simulink model "SOE_H2_DRI_plant"  (R2023b)
settings: Solver=ode15s  StartTime=0.0  StopTime=3600*24*8759
values from neighbouring files (symbols this model uses):
  a_b = 6*(1-eps_bed)/(r_p*2)    (= 200)    [H2_DRI_plant_loader.m]
  A_furnace = pi*r_furnace^2    (= 23.7582944428)    [H2_DRI_plant_loader.m]
  A_furnace_pel = A_furnace*(1-eps_bed)    (= 11.8791472214)    [H2_DRI_plant_loader.m]
  A_wall = (2*pi*r_furnace*dz)    (= 1.1674837564)    [H2_DRI_plant_loader.m]
  c_CH4init = interp1([1:1:length(c_CH4init)],c_CH4init, linspace(1,length(c_CH4init),n_furnace))    [H2_DRI_plant_loader.m]    (also in inital_conditions.m = out.CH4_conc.data(end,:); initcond_H2.mat = [9.94099064213e-45 -4.26076213273e-25 -4.27813906239e-25 -4.; initcond_H2_PEM.mat = [4.30667282687e-45 4.29087427587e-45 3.8700760922e-45 3.7994)
  c_Cinit = interp1([1:1:length(c_Cinit)],c_Cinit, linspace(1,length(c_Cinit),n_furnace))    [H2_DRI_plant_loader.m]    (also in inital_conditions.m = out.C_conc.data(end,:); initcond_H2.mat = [1.45956980986e-305 6.99081092012e-307 8.03725154841e-309 -3; initcond_H2_PEM.mat = [1.92191536232e-321 1.91203404941e-321 1.97132192691e-321 1.)
  c_CO2init = interp1([1:1:length(c_CO2init)],c_CO2init, linspace(1,length(c_CO2init),n_furnace))    [H2_DRI_plant_loader.m]    (also in inital_conditions.m = out.CO2_conc.data(end,:); initcond_H2.mat = [1.40671287015e-53 9.99429922421e-25 1.00349747704e-24 1.007; initcond_H2_PEM.mat = [4.30579616214e-45 4.28998535938e-45 3.86916279543e-45 3.798)
  c_COinit = interp1([1:1:length(c_COinit)],c_COinit, linspace(1,length(c_COinit),n_furnace))    [H2_DRI_plant_loader.m]    (also in inital_conditions.m = out.CO_conc.data(end,:); initcond_H2.mat = [8.62168160047e-54 2.62488347241e-25 2.63562031881e-25 2.646; initcond_H2_PEM.mat = [-1.41770643933e-43 -1.41248114323e-43 -1.27321677334e-43 -1)
  c_Fe2O3init = interp1([1:1:length(c_Fe2O3init)],c_Fe2O3init, linspace(1,length(c_Fe2O3init),n_furnace))    [H2_DRI_plant_loader.m]    (also in inital_conditions.m = out.Fe2O3_conc.data(end,:); initcond_H2.mat = [-0.0576294325141 -0.0562977053664 -0.0549879883395 -0.05369; initcond_H2_PEM.mat = [-0.0421766495112 -0.0410731169681 -0.0399918101679 -0.03893)
  c_Fe3O4init = interp1([1:1:length(c_Fe3O4init)],c_Fe3O4init, linspace(1,length(c_Fe3O4init),n_furnace))    [H2_DRI_plant_loader.m]    (also in inital_conditions.m = out.Fe3O4_conc.data(end,:); initcond_H2.mat = [0.0460784397936 0.0452182842983 0.0443654100081 0.043519007; initcond_H2_PEM.mat = [0.0345314201173 0.0338401633931 0.0331554273597 0.032476466)
  c_Feinit = interp1([1:1:length(c_Feinit)],c_Feinit, linspace(1,length(c_Feinit),n_furnace))    [H2_DRI_plant_loader.m]    (also in inital_conditions.m = out.Fe_conc.data(end,:); initcond_H2.mat = [2291.15615825 2257.57098555 2219.35021937 2176.85237423 213; initcond_H2_PEM.mat = [2291.15370188 2257.40533074 2219.07663621 2176.56351656 213)
  c_FeOinit = interp1([1:1:length(c_FeOinit)],c_FeOinit, linspace(1,length(c_FeOinit),n_furnace))    [H2_DRI_plant_loader.m]    (also in inital_conditions.m = out.FeO_conc.data(end,:); initcond_H2.mat = [120.587032003 163.793602795 212.96382844 267.636483226 327.; initcond_H2_PEM.mat = [120.587036941 164.003608886 213.312732219 268.005087273 327)
  c_H2init = interp1([1:1:length(c_H2init)],c_H2init, linspace(1,length(c_H2init),n_furnace))    [H2_DRI_plant_loader.m]    (also in inital_conditions.m = out.H2_conc.data(end,:); initcond_H2.mat = [22.889073739 22.8842667021 22.8746324515 22.8599710419 22.8; initcond_H2_PEM.mat = [17.1469199078 17.1645959742 17.1787956185 17.1891948084 17.)
  c_H2Oinit = interp1([1:1:length(c_H2Oinit)],c_H2Oinit, linspace(1,length(c_H2Oinit),n_furnace))    [H2_DRI_plant_loader.m]    (also in inital_conditions.m = out.H2O_conc.data(end,:); initcond_H2.mat = [2.19324064628 2.2939246227 2.40633645516 2.52967076126 2.66; initcond_H2_PEM.mat = [0.652099757837 0.728496202531 0.813916572535 0.907739128718)
  c_N2init = interp1([1:1:length(c_N2init)],c_N2init, linspace(1,length(c_N2init),n_furnace))    [H2_DRI_plant_loader.m]    (also in inital_conditions.m = out.N2_conc.data(end,:); initcond_H2.mat = [0.439764167248 0.441445162144 0.443247144888 0.445152489232; initcond_H2_PEM.mat = [0.271051060899 0.272483637209 0.274000693264 0.275587826454)
  cCarbon = 180/1000    (= 0.18)    [H2_DRI_plant_loader.m]
  CCcomp = 6151202*Pcomp^0.71    (= 33253176.5742)    [H2_DRI_plant_loader.m]
  CCeaf = 160*ls_prod_kg*8760/1000    (= 151726003.2)    [H2_DRI_plant_loader.m]
  CCelect = CC_elect*MWelect*1000    (= 480904000)    [H2_DRI_plant_loader.m]
  CCfur = 228860*Qfurnace^0.7848    (= 4163876.6695)    [H2_DRI_plant_loader.m]
  CCpsa = 30622*m_O2^0.6357    (= 6771939.09833)    [H2_DRI_plant_loader.m]
  CCsf = 250*ls_prod_kg*8760/1000    (= 237071880)    [H2_DRI_plant_loader.m]
  cLime = 100/1000    (= 0.1)    [H2_DRI_plant_loader.m]
  cNG = 7    [H2_DRI_plant_loader.m]
  CO2_diff_prop = [MM_CO2, 26.9]    [H2_DRI_plant_loader.m]
  CO_diff_prop = [MM_CO, 18.9]    [H2_DRI_plant_loader.m]
  D_metal = 0.5*I_metal    (= -0.0319284802043)    [H2_DRI_plant_loader.m]
  DRIsteel_conv = 1.075    [H2_DRI_plant_loader.m]
  dz = (h_furnace/(n_furnace-1))    (= 0.0675675675676)    [H2_DRI_plant_loader.m]
  EAF_elec_req = 375    [H2_DRI_plant_loader.m]
  eps_bed = 0.5    [H2_DRI_plant_loader.m]
  eta_comb = 0.8    [H2_DRI_plant_loader.m]
  eta_isen = 0.75    [H2_DRI_plant_loader.m]
  eta_motor = 0.95    [H2_DRI_plant_loader.m]
  H2_diff_prop = [MM_H2, 2.31*2]    [H2_DRI_plant_loader.m]
  H2O_diff_prop = [MM_H2O, 13.1]    [H2_DRI_plant_loader.m]
  H2only = true    [H2_DRI_plant_loader.m]
  hot_standby_eff = 0.009    [H2_DRI_plant_loader.m]
  I_metal = P_metal/tau_metal    (= -0.0638569604087)    [H2_DRI_plant_loader.m]
  Kd = 0.00728    [H2_DRI_plant_loader.m]
  Kmetal = -0.0435    [H2_DRI_plant_loader.m]
  labor_cost = 19*DRI_prod_kg/3600/1000 + 53*ls_prod_kg/3600/1000    (= 2.20779)    [H2_DRI_plant_loader.m]
  m_O2rate = 45.072    [H2_DRI_plant_loader.m]
  MM_C = 12.011/1000    (= 0.012011)    [H2_DRI_plant_loader.m]
  MM_CH4 = 16.04    [H2_DRI_plant_loader.m]
  MM_CO = 28.01    [H2_DRI_plant_loader.m]
  MM_CO2 = 44.01    [H2_DRI_plant_loader.m]
  MM_Fe = 55.845/1000    (= 0.055845)    [H2_DRI_plant_loader.m]    (also in iron_props.m)
  MM_Fe2O3 = 159.69/1000    (= 0.15969)    [H2_DRI_plant_loader.m]    (also in iron_props.m)
  MM_Fe3O4 = 231.53/1000    (= 0.23153)    [H2_DRI_plant_loader.m]    (also in iron_props.m = 0.25153)
  MM_FeO = 71.844/1000    (= 0.071844)    [H2_DRI_plant_loader.m]    (also in iron_props.m)
  MM_H2 = 2.016    [H2_DRI_plant_loader.m]
  MM_H2O = 18.015    [H2_DRI_plant_loader.m]
  MM_N2 = 28.013    [H2_DRI_plant_loader.m]
  MWelect = 240.452    [H2_DRI_plant_loader.m]
  MWhNGeaf = 0.08792    [H2_DRI_plant_loader.m]
  n_furnace = 75    [H2_DRI_plant_loader.m]
  ndot_H2O_feed = linspace(35, 155, n_loops)    [RTO_model_datapoints.m]
  ndot_path = ndot_path(:,3)    [H2_DRI_plant_loader.m]
  ndotin = 2706    [H2_DRI_plant_loader.m]
  nr1init = interp1([1:1:length(nr1init)],nr1init, linspace(1,length(nr1init),n_furnace))    [H2_DRI_plant_loader.m]    (also in inital_conditions.m = out.nr1.data(end,:); initcond_H2.mat = [17138.9259823 17138.9192887 17138.9127057 17138.9062259 171; initcond_H2_PEM.mat = [17138.8483125 17138.8427658 17138.8373309 17138.8319998 171)
  nr2init = interp1([1:1:length(nr2init)],nr2init, linspace(1,length(nr2init),n_furnace))    [H2_DRI_plant_loader.m]    (also in inital_conditions.m = out.nr2.data(end,:); initcond_H2.mat = [11425.7909148 11425.7894343 11425.7880023 11425.7866166 114; initcond_H2_PEM.mat = [11425.7791649 11425.7778635 11425.776614 11425.7754137 1142)
  nr3init = interp1([1:1:length(nr3init)],nr3init, linspace(1,length(nr3init),n_furnace))    [H2_DRI_plant_loader.m]    (also in inital_conditions.m = out.nr3.data(end,:); initcond_H2.mat = [32930.1678524 32447.4572478 31898.1205118 31287.3104766 306; initcond_H2_PEM.mat = [32930.1325476 32445.0763361 31894.188375 31283.1588034 3061)
  oxy_eff_tonne = 0.803    [H2_DRI_plant_loader.m]
  P_g_sp = 101325*2.5    (= 253312.5)    [H2_DRI_plant_loader.m]
  P_metal = tau_metal/(Kmetal*tau_metal_desired)    (= -735.632183908)    [H2_DRI_plant_loader.m]
  pandcdata = csvread('caiso_lmp_carbon_clean.csv', 1, 1)    [H2_DRI_plant_loader.m]
  R = 8.314    [Bou.m]    (also in H2_DRI_plant_loader.m; MD.m; SMR.m; USCM_CO.m)
  r_furnace = 2.75    [H2_DRI_plant_loader.m]
  r_p = 15e-3/2    (= 0.0075)    [H2_DRI_plant_loader.m]
  rho_p = 3528    [H2_DRI_plant_loader.m]
  SOEeff = 37.5    [H2_DRI_plant_loader.m]
  stack_replace = 3.25    [H2_DRI_plant_loader.m]
  T_gin = 950 + 273    (= 1223)    [H2_DRI_plant_loader.m]
  T_ginit = interp1([1:1:length(T_ginit)],T_ginit, linspace(1,length(T_ginit),n_furnace))    [H2_DRI_plant_loader.m]    (also in inital_conditions.m = out.T_g.data(end,2:end); initcond_H2.mat = [1193.47241077 1188.60147936 1183.4413554 1178.04610025 1172; initcond_H2_PEM.mat = [1213.62674902 1206.86882145 1199.80656651 1192.51337179 118)
  T_sin = 10 + 273    (= 283)    [H2_DRI_plant_loader.m]
  T_sinit = interp1([1:1:length(T_sinit)],T_sinit, linspace(1,length(T_sinit),n_furnace))    [H2_DRI_plant_loader.m]    (also in inital_conditions.m = out.T_s.data(end,1:end-1); initcond_H2.mat = [1188.32225462 1183.11411515 1177.66723955 1172.0331792 1166; initcond_H2_PEM.mat = [1207.76768382 1200.67884676 1193.34151616 1185.82650883 117)
  tau = 1    [H2_DRI_plant_loader.m]
  tau_d = 3600    [H2_DRI_plant_loader.m]
  tau_metal = 3.2*3600    (= 11520)    [H2_DRI_plant_loader.m]
  taxes = tax_rate*TIC/8760/3600    [H2_DRI_plant_loader.m]
  V_g = (4/3)*pi*r_p^3*n_pellets_dz*(eps_bed/(1-eps_bed))    (= 0.802645082526)    [H2_DRI_plant_loader.m]
  V_p = 4/3*pi*r_p^3    (= 1.76714586764e-06)    [H2_DRI_plant_loader.m]
  V_s = (4/3)*pi*r_p^3*n_pellets_dz    (= 0.802645082526)    [H2_DRI_plant_loader.m]
  w_Cin = 0    [H2_DRI_plant_loader.m]
  w_Fe2O3in = 0.9665    [H2_DRI_plant_loader.m]
  w_Fe3O4in = 0    [H2_DRI_plant_loader.m]
  w_Fein = 0    [H2_DRI_plant_loader.m]
  w_FeOin = 0    [H2_DRI_plant_loader.m]
  w_Ganin = 0.0335    [H2_DRI_plant_loader.m]
  x_H2in = 0.90    (= 0.9)    [H2_DRI_plant_loader.m]
  x_H2Oin = 0.085    [H2_DRI_plant_loader.m]
  x_N2in = 0.015    [H2_DRI_plant_loader.m]
undefined symbols (not defined in the file or in its folder): CCbop
libraries: slpidlib x2
(part 1 of 3)
settings Model: Creator=jimmonen  LastModifiedBy=jimmonen
settings SolverCC: ZeroCrossAlgorithm=Adaptive  AlgebraicLoopSolver=TrustRegion
settings DebuggingCC: IgnoredZcDiagnostic=none  UnconnectedInputMsg=warning  UnconnectedOutputMsg=warning  UnconnectedLineMsg=warning
settings ModelReferenceCC: EnableRefExpFcnMdlSchedulingChecks=on
settings RTWCC: DLArmComputeVersion=19.05

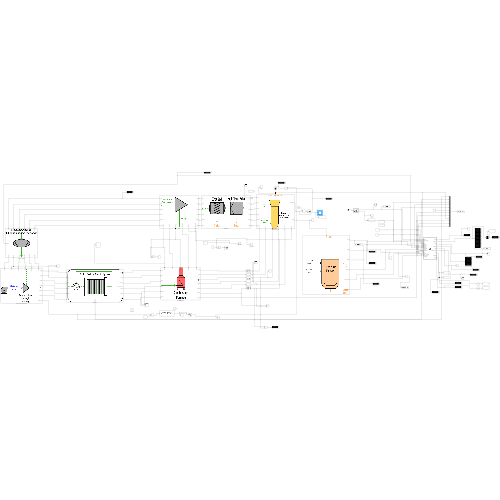
[thumbnail: Simulink's stored preview of the top-level diagram]
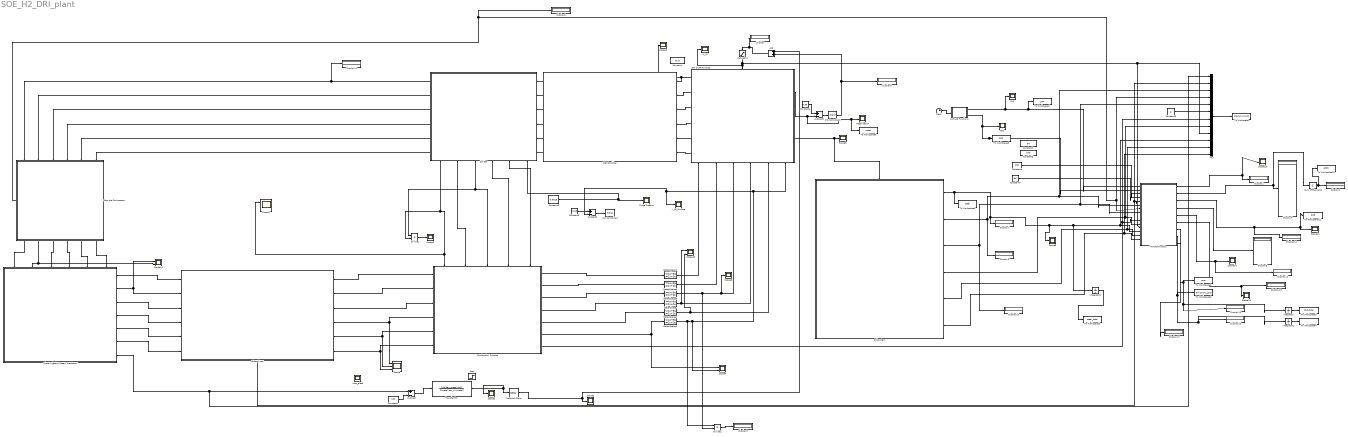
== system SOE_H2_DRI_plant ==
  Add : Sum
  CO2 : Scope
  Clock : Clock
  Combustion Furnace : Subsystem
      settings: PortSchema="{\"entries\":[{\"content\":{\"sides\":[{\"content\":{\"connectorIds\":[\"In1\",\"In2\",\"In3\",\"In4\",\"In5\",\"In6\"]},\"type\":\"ConnectorPlacement.EquallySpacedRectSide\",\"uuid\":\"8f0827ee-30e7-4902-8795-b9cbf5da36d9\"},{\"content\":{\"connectorIds\":[\"Out1\",\"Out2\",\"Out3\",\"Out4\",\"Out5\",\"Out6\",\"Out7\"],\"side\":\"RIGHT\"},\"type\":\"ConnectorPlacement.EquallySpacedRectSide\",\"uuid\":\"60662037-2ede-4f16-84f2-d3e372a712be\"},{\"content\":{\"connectorIds\":[\"In7\",\"In8\",\"In9\",\"In10\",\"In11\"],\"side\":\"TOP\"},\"type\":\"ConnectorPlacement.EquallySpacedRectSide\",\"uuid\":\"a8014c68-6626-4e3b-a233-1219219a26e0\"},{\"content\":{\"connectorIds\":[\"In12\"],\"side\":\"BOTTOM\"},\"type\":\"ConnectorPlacement.EquallySpacedRectSide\",\"uuid\":\"bb3bbeea-0196-4549-b4fc-2f2ced4efafc\"}]},\"type\":\"ConnectorPlacement.EquallySpacedConnector\",\"uuid\":\"c7227bf4-9e67-4938-bab2-cc4a9329a3cb\"}],\"packageUris\":[\"http://schema.mathworks.com/mf0/Connector/R2020b\"],\"version\":\"1.0\"}"
      mask Display: image('Comb Furnace.drawio.png');
  Constant : Constant  Value=41.8
  Constant1 : Constant  Value=150
  Constant2 : Constant  Value=84
  Constant3 : Constant  Value=0.015
  Constant4 : Constant  Value=0.95
  Constant5 : Constant  Value=100
  Constant6 : Constant  Value=130
  Constant7 : Constant  Value=847
  Constant8 : Constant  Value=0.0615
  Constant9 : Constant  Value=0
  DRI Shaft Furnace : Subsystem
      settings: PortSchema="{\"entries\":[{\"content\":{\"sides\":[{\"content\":{\"connectorIds\":[\"Out7\",\"Out8\"]},\"type\":\"ConnectorPlacement.EquallySpacedRectSide\",\"uuid\":\"924f0eb5-1be8-4fbc-81da-68f87f043754\"},{\"content\":{\"connectorIds\":[\"Out1\",\"Out2\",\"Out3\",\"Out4\",\"Out5\",\"Out6\"],\"side\":\"RIGHT\"},\"type\":\"ConnectorPlacement.EquallySpacedRectSide\",\"uuid\":\"1615a0ab-d9ff-4201-ad7d-89e25dee6d75\"},{\"content\":{\"connectorIds\":[\"In1\"],\"side\":\"TOP\"},\"type\":\"ConnectorPlacement.EquallySpacedRectSide\",\"uuid\":\"9aa5edee-f4b9-4baa-b28d-7fcf4cc3e066\"},{\"content\":{\"connectorIds\":[\"In2\",\"In3\",\"In4\",\"In5\",\"In6\",\"In7\"],\"side\":\"BOTTOM\"},\"type\":\"ConnectorPlacement.EquallySpacedRectSide\",\"uuid\":\"9b247e36-6ea5-4bcc-bfed-c8482ad4e5f5\"}]},\"type\":\"ConnectorPlacement.EquallySpacedConnector\",\"uuid\":\"df526a9b-01b4-44b1-91cd-061142fed636\"}],\"packageUris\":[\"http://schema.mathworks.com/mf0/Connector/R2020b\"],\"version\":\"1.0\"}"
      mask Display: image('DRI Shaft Furnace.drawio.png');
  Direct Injection Steam Generator : Subsystem
      settings: PortSchema="{\"entries\":[{\"content\":{\"sides\":[{\"content\":{},\"type\":\"ConnectorPlacement.EquallySpacedRectSide\",\"uuid\":\"655e84cb-69cf-4761-b101-58ad49abce33\"},{\"content\":{\"connectorIds\":[\"Out1\",\"Out2\",\"Out3\",\"Out4\",\"Out5\",\"Out6\",\"Out7\"],\"side\":\"RIGHT\"},\"type\":\"ConnectorPlacement.EquallySpacedRectSide\",\"uuid\":\"c22001c3-4fe9-4ca1-8f86-27c8b9cf3215\"},{\"content\":{\"connectorIds\":[\"In1\",\"In2\",\"In3\",\"In4\",\"In5\",\"In6\"],\"side\":\"TOP\"},\"type\":\"ConnectorPlacement.EquallySpacedRectSide\",\"uuid\":\"85460019-312d-4580-833a-9195b760a2b2\"}]},\"type\":\"ConnectorPlacement.EquallySpacedConnector\",\"uuid\":\"a09837c3-5ba4-4c5d-b1a3-49fb7b0895f7\"}],\"packageUris\":[\"http://schema.mathworks.com/mf0/Connector/R2020b\"],\"version\":\"1.0\"}"
      mask Display: image('DRI Plants-evaporator.drawio.png');
  Display{,1..17} (18 alike) : Display
  Divide1 : Product  Inputs=**
  Divide2 : Product  Inputs=**
  Electrolyzer : Subsystem
      settings: PortSchema="{\"entries\":[{\"content\":{\"sides\":[{\"content\":{\"connectorIds\":[\"In1\",\"In2\",\"In3\",\"In4\",\"In5\",\"In6\"]},\"type\":\"ConnectorPlacement.EquallySpacedRectSide\",\"uuid\":\"236efb1b-599d-46dd-879b-994191023a3b\"},{\"content\":{\"connectorIds\":[\"Out1\",\"Out2\",\"Out3\",\"Out4\",\"Out5\",\"Out6\"],\"side\":\"RIGHT\"},\"type\":\"ConnectorPlacement.EquallySpacedRectSide\",\"uuid\":\"4fb8c9ef-fe44-4b5c-925a-977108b57150\"},{\"content\":{\"side\":\"TOP\"},\"type\":\"ConnectorPlacement.EquallySpacedRectSide\",\"uuid\":\"6a10da36-9c65-49c1-b0b0-73c6f2698fc8\"},{\"content\":{\"connectorIds\":[\"Out7\"],\"side\":\"BOTTOM\"},\"type\":\"ConnectorPlacement.EquallySpacedRectSide\",\"uuid\":\"5907bdd8-7e1e-4fa5-8f12-20141da20536\"}]},\"type\":\"ConnectorPlacement.EquallySpacedConnector\",\"uuid\":\"599bc2dd-5d5b-4fb1-b91a-53aceb0c006b\"}],\"packageUris\":[\"http://schema.mathworks.com/mf0/Connector/R2020b\"],\"version\":\"1.0\"}"
      mask Display: image('DRI Plants-SOE.drawio.png');
  Integrator : Integrator
  Integrator1 : Integrator
  Integrator2 : Integrator
  LMP : Scope
  MATLAB Function : MATLAB Function  TreatAsAtomicUnit=on
  MATLAB Function1 : MATLAB Function  TreatAsAtomicUnit=on
  Metallization : Scope
  Mux : Mux  Inputs=12
  PID Controller1 : slpidlib/PID Controller  Controller=PID  Form=Parallel  TimeDomain=Continuous-time  UseExternalTs=off  SampleTime=-1  IntegratorMethod=Forward Euler  FilterMethod=Forward Euler  ControllerParametersSource=internal  P=-10  I=-0.0069  UseKiTs=off  D=0  N=100  UseFilter=on  TunerSelectOption=Transfer Function Based (PID Tuner App)  InitialConditionSource=internal  InitialConditionForIntegrator=0.065  InitialConditionForFilter=0.065  DifferentiatorICPrevScaledInput=0  ExternalReset=none  TrackingMode=off  Kt=1  LimitOutput=on  SatLimitsSource=internal  UpperSaturationLimit=0.08  LowerSaturationLimit=0.05  LinearizeAsGain=on  AntiWindupMode=clamping  Kb=1  LimitIntegrator=off  UpperIntegratorSaturationLimit=inf  LowerIntegratorSaturationLimit=-inf  POutMin=[]  POutMax=[]  IOutMin=[]  IOutMax=[]  DOutMin=[]  DOutMax=[]  NOutMin=[]  NOutMax=[]  SumOutMin=[]  SumOutMax=[]  SaturationOutMin=[]  SaturationOutMax=[]  PParamMin=[]  PParamMax=[]  IParamMin=[]  IParamMax=[]  DParamMin=[]  DParamMax=[]  NParamMin=[]  NParamMax=[]  KbParamMin=[]  KbParamMax=[]  KtParamMin=[]  KtParamMax=[]  KbOutMin=[]  KbOutMax=[]  KtOutMin=[]  KtOutMax=[]  IntegratorOutMin=[]  IntegratorOutMax=[]  FilterOutMin=[]  FilterOutMax=[]  SumI1OutMin=[]  SumI1OutMax=[]  SumI2OutMin=[]  SumI2OutMax=[]  SumI3OutMin=[]  SumI3OutMax=[]  SumI4OutMin=[]  SumI4OutMax=[]  SumDOutMin=[]  SumDOutMax=[]  DifferentiatorOutMin=[]  DifferentiatorOutMax=[]  FilterDiffOutCoefMin=[]  FilterDiffOutCoefMax=[]  ReciprocalOutMin=[]  ReciprocalOutMax=[]  SumDenOutMin=[]  SumDenOutMax=[]  SumNumOutMin=[]  SumNumOutMax=[]  DivideOutMin=[]  DivideOutMax=[]  UdiffTsProdOutMin=[]  UdiffTsProdOutMax=[]  NTsProdOutMin=[]  NTsProdOutMax=[]  UintegralTsProdOutMin=[]  UintegralTsProdOutMax=[]  UngainTsProdOutMin=[]  UngainTsProdOutMax=[]  ClampingZeroOutDataTypeStr=Inherit: Inherit via back propagation  ClampingZeroOutMin=[]  ClampingZeroOutMax=[]  FilterDenConstantOutDataTypeStr=Inherit: Inherit via back propagation  FilterDenConstantOutMin=[]  FilterDenConstantOutMax=[]  PCopyOutDataTypeStr=Inherit: Inherit via back propagation  PCopyOutMin=[]  PCopyOutMax=[]  NCopyOutDataTypeStr=Inherit: Inherit via back propagation  NCopyOutMin=[]  NCopyOutMax=[]  IntegratorContinuousStateAttributes=''  IntegratorStateMustResolveToSignalObject=off  IntegratorRTWStateStorageClass=Auto  FilterContinuousStateAttributes=''  FilterStateMustResolveToSignalObject=off  FilterRTWStateStorageClass=Auto  ParallelPVariant=InternalParameters  IdealPVariant=Disabled  IVariant=InternalParameters  DVariant=InternalParameters  IntegratorVariant=Continuous  SatVariant=Enabled  AWVariant=ContClampingParallel  PCopyVariant=Disabled  TRVariant=Disabled  FdbkBlocksVariant=Forward  IdealPFdbkVariant=Disabled  SatFdbkVariant=Disabled  DerivativeFilterVariant=ContFilter  NVariant=InternalParameters  NCopyVariant=Disabled  FilterICVariant=InternalICsFilter  IntegratorICVariant=InternalICs  ExternalResetVariant=Disabled  TRSumVariant=Passthrough  SumFdbkVariant=Disabled  SumVariant=Sum_PID  TsampFilterVariant=InternalTs  TsampNgainVariant=Passthrough  TsampIntegralVariant=Disabled_SignalSpec  ExternalSaturationOutDataTypeStr=Inherit: Same as second input
  PID Controller2 : slpidlib/PID Controller  Controller=PID  Form=Parallel  TimeDomain=Continuous-time  UseExternalTs=off  SampleTime=-1  IntegratorMethod=Forward Euler  FilterMethod=Forward Euler  ControllerParametersSource=internal  P=P_metal  I=I_metal  UseKiTs=off  D=D_metal  N=100  UseFilter=on  TunerSelectOption=Transfer Function Based (PID Tuner App)  ZeroCross=off  InitialConditionSource=internal  InitialConditionForIntegrator=45  InitialConditionForFilter=45  DifferentiatorICPrevScaledInput=0  ExternalReset=none  TrackingMode=off  Kt=1  LimitOutput=on  SatLimitsSource=internal  UpperSaturationLimit=60  LowerSaturationLimit=10  LinearizeAsGain=on  AntiWindupMode=clamping  Kb=1  LimitIntegrator=off  UpperIntegratorSaturationLimit=inf  LowerIntegratorSaturationLimit=-inf  POutMin=[]  POutMax=[]  IOutMin=[]  IOutMax=[]  DOutMin=[]  DOutMax=[]  NOutMin=[]  NOutMax=[]  SumOutMin=[]  SumOutMax=[]  SaturationOutMin=[]  SaturationOutMax=[]  PParamMin=[]  PParamMax=[]  IParamMin=[]  IParamMax=[]  DParamMin=[]  DParamMax=[]  NParamMin=[]  NParamMax=[]  KbParamMin=[]  KbParamMax=[]  KtParamMin=[]  KtParamMax=[]  KbOutMin=[]  KbOutMax=[]  KtOutMin=[]  KtOutMax=[]  IntegratorOutMin=[]  IntegratorOutMax=[]  FilterOutMin=[]  FilterOutMax=[]  SumI1OutMin=[]  SumI1OutMax=[]  SumI2OutMin=[]  SumI2OutMax=[]  SumI3OutMin=[]  SumI3OutMax=[]  SumI4OutMin=[]  SumI4OutMax=[]  SumDOutMin=[]  SumDOutMax=[]  DifferentiatorOutMin=[]  DifferentiatorOutMax=[]  FilterDiffOutCoefMin=[]  FilterDiffOutCoefMax=[]  ReciprocalOutMin=[]  ReciprocalOutMax=[]  SumDenOutMin=[]  SumDenOutMax=[]  SumNumOutMin=[]  SumNumOutMax=[]  DivideOutMin=[]  DivideOutMax=[]  UdiffTsProdOutMin=[]  UdiffTsProdOutMax=[]  NTsProdOutMin=[]  NTsProdOutMax=[]  UintegralTsProdOutMin=[]  UintegralTsProdOutMax=[]  UngainTsProdOutMin=[]  UngainTsProdOutMax=[]  ClampingZeroOutDataTypeStr=Inherit: Inherit via back propagation  ClampingZeroOutMin=[]  ClampingZeroOutMax=[]  FilterDenConstantOutDataTypeStr=Inherit: Inherit via back propagation  FilterDenConstantOutMin=[]  FilterDenConstantOutMax=[]  PCopyOutDataTypeStr=Inherit: Inherit via back propagation  PCopyOutMin=[]  PCopyOutMax=[]  NCopyOutDataTypeStr=Inherit: Inherit via back propagation  NCopyOutMin=[]  NCopyOutMax=[]  IntegratorContinuousStateAttributes=''  IntegratorStateMustResolveToSignalObject=off  IntegratorRTWStateStorageClass=Auto  FilterContinuousStateAttributes=''  FilterStateMustResolveToSignalObject=off  FilterRTWStateStorageClass=Auto  ParallelPVariant=InternalParameters  IdealPVariant=Disabled  IVariant=InternalParameters  DVariant=InternalParameters  IntegratorVariant=Continuous  SatVariant=Enabled  AWVariant=ContClampingParallel  PCopyVariant=Disabled  TRVariant=Disabled  FdbkBlocksVariant=Forward  IdealPFdbkVariant=Disabled  SatFdbkVariant=Disabled  DerivativeFilterVariant=ContFilter  NVariant=InternalParameters  NCopyVariant=Disabled  FilterICVariant=InternalICsFilter  IntegratorICVariant=InternalICs  ExternalResetVariant=Disabled  TRSumVariant=Passthrough  SumFdbkVariant=Disabled  SumVariant=Sum_PID  TsampFilterVariant=InternalTs  TsampNgainVariant=Passthrough  TsampIntegralVariant=Disabled_SignalSpec  ExternalSaturationOutDataTypeStr=Inherit: Same as second input
  Purge Fraction : Scope
  Recycle Compressor : Subsystem
      settings: PortSchema="{\"entries\":[{\"content\":{\"sides\":[{\"content\":{\"connectorIds\":[\"In1\",\"In2\",\"In3\",\"In4\",\"In5\",\"In6\"]},\"type\":\"ConnectorPlacement.EquallySpacedRectSide\",\"uuid\":\"a27e49e6-5f88-4807-8689-82055264f808\"},{\"content\":{\"connectorIds\":[\"Out1\",\"Out2\",\"Out3\",\"Out4\",\"Out5\",\"Out6\"],\"side\":\"RIGHT\"},\"type\":\"ConnectorPlacement.EquallySpacedRectSide\",\"uuid\":\"3c1e61fb-ea44-4a9f-bafc-cf85fd83c3b0\"},{\"content\":{\"connectorIds\":[\"Out7\"],\"side\":\"TOP\"},\"type\":\"ConnectorPlacement.EquallySpacedRectSide\",\"uuid\":\"024adc8a-c386-4dd0-b22e-90eb96d1d83c\"}]},\"type\":\"ConnectorPlacement.EquallySpacedConnector\",\"uuid\":\"5bc88750-df40-472f-99b3-d87672963f0a\"}],\"packageUris\":[\"http://schema.mathworks.com/mf0/Connector/R2020b\"],\"version\":\"1.0\"}"
      mask Display: image('Recycle Comp.drawio.png');
  Saturation : Saturate  UpperLimit=60  LowerLimit=10
  Scope : Scope  NumInputPorts=3
  Scope{1..3,5..6,8..11,14..15} (11 alike) : Scope
  Scope{4,7,12..13} (4 alike) : Scope  NumInputPorts=2
  Splitter : Subsystem
      settings: PortSchema="{\"entries\":[{\"content\":{\"sides\":[{\"content\":{\"connectorIds\":[\"In1\",\"In2\",\"In3\",\"In4\",\"In5\",\"In6\"]},\"type\":\"ConnectorPlacement.EquallySpacedRectSide\",\"uuid\":\"fd25b217-e1f0-4070-96cf-364215ce8118\"},{\"content\":{\"connectorIds\":[\"Out1\",\"Out2\",\"Out3\",\"Out4\",\"Out5\",\"Out6\"],\"side\":\"RIGHT\"},\"type\":\"ConnectorPlacement.EquallySpacedRectSide\",\"uuid\":\"2bc1ddce-05b6-409e-8141-f4e0eb59e520\"},{\"content\":{\"side\":\"TOP\"},\"type\":\"ConnectorPlacement.EquallySpacedRectSide\",\"uuid\":\"93ff0178-d151-4804-b3d4-a05ee4ee5065\"},{\"content\":{\"connectorIds\":[\"In7\",\"Out7\",\"Out8\",\"Out9\",\"Out10\",\"Out11\"],\"side\":\"BOTTOM\"},\"type\":\"ConnectorPlacement.EquallySpacedRectSide\",\"uuid\":\"a0b3f245-88e8-4c4e-8824-c9c2fceba87f\"}]},\"type\":\"ConnectorPlacement.EquallySpacedConnector\",\"uuid\":\"398b79cc-d110-4656-88d4-fd64d4a6558b\"}],\"packageUris\":[\"http://schema.mathworks.com/mf0/Connector/R2020b\"],\"version\":\"1.0\"}"
      mask Display: image('splitter.drawio.png');
  State-Space : StateSpace  A=-1/(tau)  B=1/(tau)  D=0  InitialCondition=x_H2in
  State-Space2 : StateSpace  A=-1/(tau)  B=1/(tau)  D=0  InitialCondition=x_H2Oin
  State-Space3 : StateSpace  A=-1/(tau)  B=1/(tau)  D=0  InitialCondition=x_N2in
  State-Space6 : StateSpace  A=-1/(tau)  B=1/(tau)  D=0  InitialCondition=ndotin
  State-Space7 : StateSpace  A=-1/(tau)  B=1/(tau)  D=0  InitialCondition=P_g_sp
  State-Space8 : StateSpace  A=-1/(tau)  B=1/(tau)  D=0  InitialCondition=T_gin
  Step : Step  Time=3600*24  Before=T_gin  After=T_gin-100  SampleTime=0
  Subsystem : Subsystem
      settings: PortSchema="{\"entries\":[{\"content\":{\"sides\":[{\"content\":{},\"type\":\"ConnectorPlacement.EquallySpacedRectSide\",\"uuid\":\"a5720816-84e5-4a89-90be-c62fc29b155a\"},{\"content\":{\"connectorIds\":[\"Out1\",\"Out2\",\"Out3\",\"Out4\",\"Out5\",\"Out6\"],\"side\":\"RIGHT\"},\"type\":\"ConnectorPlacement.EquallySpacedRectSide\",\"uuid\":\"f64801c4-e566-4939-8d57-f551d182a2a2\"},{\"content\":{\"connectorIds\":[\"In1\"],\"side\":\"TOP\"},\"type\":\"ConnectorPlacement.EquallySpacedRectSide\",\"uuid\":\"024857d9-9643-47ab-98d7-ab5b369169d3\"}]},\"type\":\"ConnectorPlacement.EquallySpacedConnector\",\"uuid\":\"93b03b57-3aff-49fd-8d1e-5b59ac681d1d\"}],\"packageUris\":[\"http://schema.mathworks.com/mf0/Connector/R2020b\"],\"version\":\"1.0\"}"
      mask Display: image('EAF.drawio.png');
  Subtract : Sum  Inputs=+-
  Subtract1 : Sum  Inputs=+-
  Subtract2 : Sum  Inputs=+-
  Sum of Elements : Sum  Inputs=+
  To Workspace : ToWorkspace  VariableName=obj_fun_inputs  SaveFormat=Timeseries  SampleTime=-1
  To Workspace1 : ToWorkspace  VariableName=cost  SaveFormat=Timeseries  SampleTime=-1
  To Workspace10 : ToWorkspace  VariableName=LCOS  SaveFormat=Timeseries  SampleTime=-1
  To Workspace11 : ToWorkspace  VariableName=SCE  SaveFormat=Timeseries  SampleTime=-1
  To Workspace2 : ToWorkspace  VariableName=emissions_cost  SaveFormat=Timeseries  SampleTime=-1
  To Workspace3 : ToWorkspace  VariableName=cost_total  SaveFormat=Timeseries  SampleTime=-1
  To Workspace4 : ToWorkspace  VariableName=emissions_cost_total  SaveFormat=Timeseries  SampleTime=-1
  To Workspace5 : ToWorkspace  VariableName=steel_total  SaveFormat=Timeseries  SampleTime=-1
  To Workspace6 : ToWorkspace  VariableName=metal  SaveFormat=Timeseries  SampleTime=-1
  To Workspace7 : ToWorkspace  VariableName=LMP  SaveFormat=Timeseries  SampleTime=-1
  To Workspace8 : ToWorkspace  VariableName=CO2  SaveFormat=Timeseries  SampleTime=-1
  To Workspace9 : ToWorkspace  VariableName=steel  SaveFormat=Timeseries  SampleTime=-1
  Transfer Fcn : TransferFcn  Numerator=[-Kd*tau_metal -Kd ]  Denominator=[Kmetal*tau_d Kmetal]
  Transport Delay : TransportDelay  DelayTime=3600/2
  Wet Scrubber : Subsystem
      mask Display: image('DRI Plants-Zn.drawio.png');
  m_IO : Scope
  ndot_elect : Scope
  x_N2_furnace : Scope
  wires:
  DRI Shaft Furnace/1(P_gout) -> Scope9/1, Wet Scrubber/1(P_gin)
  DRI Shaft Furnace/2(T_gout) -> Wet Scrubber/2(T_gin)
  DRI Shaft Furnace/4(x_H2out) -> Wet Scrubber/4(x_H2in)
  DRI Shaft Furnace/5(x_H2Oout) -> Wet Scrubber/5(x_H2Oin)
  Wet Scrubber/1(P_gout) -> Splitter/1(P_gin)
  Wet Scrubber/2(T_gout) -> Splitter/2(T_gin)
  Wet Scrubber/4(x_H2out) -> Splitter/4(x_H2in)
  Wet Scrubber/5(x_H2Oout) -> Splitter/5(x_H2Oin)
  Splitter/1(P_gout) -> Display14/1, Recycle Compressor/1(P_gin)
  Splitter/2(T_gout) -> Recycle Compressor/2(T_gin)
  Splitter/4(x_H2out) -> Recycle Compressor/4(x_H2in)
  Splitter/5(x_H2Oout) -> Recycle Compressor/5(x_H2Oin)
  Recycle Compressor/1(P_gout) -> Direct Injection Steam Generator/1(P_gin_r)
  Recycle Compressor/2(T_gout) -> Scope12/2, Direct Injection Steam Generator/2(T_gin_r)
  Recycle Compressor/4(x_H2out) -> Direct Injection Steam Generator/4(x_H2in_r)
  Recycle Compressor/5(x_H2Oout) -> Direct Injection Steam Generator/5(x_H2Oin_r)
  Direct Injection Steam Generator/2(T_gout) -> Electrolyzer/2(T_gin), Scope12/1
  Combustion Furnace/4(x_H2out) -> State-Space/1
  Combustion Furnace/5(x_H2Oout) -> State-Space2/1
  Combustion Furnace/6(x_N2out) -> State-Space3/1, Scope4/1
  Combustion Furnace/2(T_gout) -> State-Space8/1
  Combustion Furnace/3(ndot_out) -> State-Space6/1
  Combustion Furnace/1(P_gout) -> State-Space7/1
  State-Space7/1 -> DRI Shaft Furnace/7(P_gin)
  State-Space8/1 -> DRI Shaft Furnace/6(T_gin)
  State-Space/1 -> Scope13/1, DRI Shaft Furnace/4(x_H2in)
  State-Space2/1 -> Scope13/2, DRI Shaft Furnace/3(x_H2Oin)
  Subtract1/1 -> PID Controller1/1
  Constant3/1 -> Subtract1/1
  Constant8/1 -> Purge Fraction/1, Splitter/7(Purge Fraction)
  Divide2/1 -> Display3/1
  State-Space6/1 -> Divide2/2, Scope3/1, DRI Shaft Furnace/5(ndot_gin)
  DRI Shaft Furnace/6(x_N2out) -> Wet Scrubber/6(x_N2in)
  DRI Shaft Furnace/3(ndotout) -> Wet Scrubber/3(ndotin)
  Wet Scrubber/3(ndotout) -> Splitter/3(ndotin)
  Wet Scrubber/6(x_N2out) -> Splitter/6(x_N2in)
  Splitter/3(ndot_comp) -> Recycle Compressor/3(ndotin)
  Splitter/6(x_N2out) -> Recycle Compressor/6(x_N2in)
  Recycle Compressor/3(ndotout) -> Direct Injection Steam Generator/3(ndotin_r)
  Recycle Compressor/6(x_N2out) -> Direct Injection Steam Generator/6(x_N2in_r)
  State-Space3/1 -> Divide2/1, Scope4/2, x_N2_furnace/1, Subtract1/2, DRI Shaft Furnace/2(x_N2in)
  Subtract2/1 -> PID Controller2/1
  Constant4/1 -> Subtract2/1
  DRI Shaft Furnace/7(Mettalization) -> To Workspace6/1, Metallization/1, Subtract2/2
  PID Controller2/1 -> Display9/1, Add/2
  Splitter/10(T_gout_p) -> Combustion Furnace/8(T_p)
  Splitter/8(x_H2Oout_p) -> Combustion Furnace/10(x_H2O_p)
  Splitter/7(x_N2outp) -> Combustion Furnace/11(x_N2_p)
  Electrolyzer/6(x_N2out) -> Combustion Furnace/6(x_N2in), Scope/3
  Add/1 -> Saturation/1, Display/1
  Transport Delay/1 -> Add/1, Scope1/1
  Transfer Fcn/1 -> Scope2/1, Transport Delay/1
  Subtract/1 -> Transfer Fcn/1
  Constant1/1 -> Subtract/2
  DRI Shaft Furnace/8(m_DRI) -> Subsystem/1(m_DRI), Scope5/1
  Splitter/11(ndot_purge) -> Divide1/2, Scope7/1, Combustion Furnace/7(ndot_p)
  Divide1/1 -> Scope6/1
  Splitter/9(x_H2out_p) -> Divide1/1, Combustion Furnace/9(x_H2_p)
  MATLAB Function/1(LCOS) -> Scope10/1, Display1/1
  MATLAB Function/2(LCOS_bd) -> Sum of Elements/1, Display4/1
  Subsystem/2(MWeaf) -> Display8/1, Mux/3, MATLAB Function/6(MWeaf)
  Subsystem/1(m_steel) -> To Workspace9/1, Display7/1, Scope8/1, Integrator2/1, Mux/10, MATLAB Function/13(m_steel)
  Subsystem/3(MWpsa) -> Display10/1, Mux/5, MATLAB Function/8(MWpsa)
  Combustion Furnace/7(MW_ng) -> Mux/7, MATLAB Function/10(MWng)
  Subsystem/5(carbon_consume) -> Mux/11, MATLAB Function/14(carbon_consume)
  Subsystem/6(lime_consume) -> Mux/12, MATLAB Function/15(lime_consume)
  Subsystem/4(MWng_eaf) -> Mux/8, MATLAB Function/11(MWng_eaf)
  MATLAB Function/3(SCE) -> Display11/1, To Workspace11/1, Scope11/1
  MATLAB Function1/1(LCOE) -> LMP/1, To Workspace7/1, MATLAB Function/1(LCOE)
  MATLAB Function/4(SCE_bd) -> Display5/1
  Recycle Compressor/7(MWcomp) -> Display6/1, Mux/4, MATLAB Function/7(MWcomp)
  Mux/1 -> To Workspace/1
  MATLAB Function/5(profit) -> Scope14/1, Display12/1
  Constant6/1 -> MATLAB Function/3(cIO)
  Constant7/1 -> MATLAB Function/4(pLS)
  MATLAB Function/6(emissions_profit) -> Scope15/1, Display13/1
  Direct Injection Steam Generator/1(P_gout) -> Electrolyzer/1(P_gin)
  Direct Injection Steam Generator/3(ndotout) -> Electrolyzer/3(ndot_in)
  Direct Injection Steam Generator/4(x_H2out) -> Electrolyzer/4(x_H2in)
  Direct Injection Steam Generator/5(x_H2Oout) -> Electrolyzer/5(x_H2Oin)
  Direct Injection Steam Generator/6(x_N2out) -> Electrolyzer/6(x_N2in)
  Electrolyzer/1(P_gout) -> Combustion Furnace/1(P_gin)
  Electrolyzer/2(T_gout) -> Combustion Furnace/2(T_gin)
  Electrolyzer/3(ndot_out) -> Combustion Furnace/3(ndotin)
  Electrolyzer/4(x_H2out) -> Combustion Furnace/4(x_H2in), Scope/1
  Electrolyzer/5(x_H2Oout) -> Combustion Furnace/5(x_H2Oin), Scope/2
  Electrolyzer/7(MWelect) -> Mux/2, MATLAB Function/5(MWelect)
  Direct Injection Steam Generator/7(ndotH2O_mu) -> Mux/1, Subtract/1
  Constant9/1 -> Mux/6
  Saturation/1 -> MATLAB Function/12(m_IO), Mux/9, DRI Shaft Furnace/1(m_sin), m_IO/1
  Sum of Elements/1 -> To Workspace10/1, Display2/1
  MATLAB Function/7(cost) -> Integrator/1, Display15/1, To Workspace1/1
  MATLAB Function/8(emissions) -> To Workspace2/1, Integrator1/1, Display16/1
  Clock/1 -> MATLAB Function1/1(time)
  Integrator/1 -> To Workspace3/1
  Integrator1/1 -> To Workspace4/1
  Integrator2/1 -> To Workspace5/1
  MATLAB Function/9(MWe) -> Display17/1
  MATLAB Function1/2(CO2) -> CO2/1, MATLAB Function/2(elec_CO2rate), To Workspace8/1

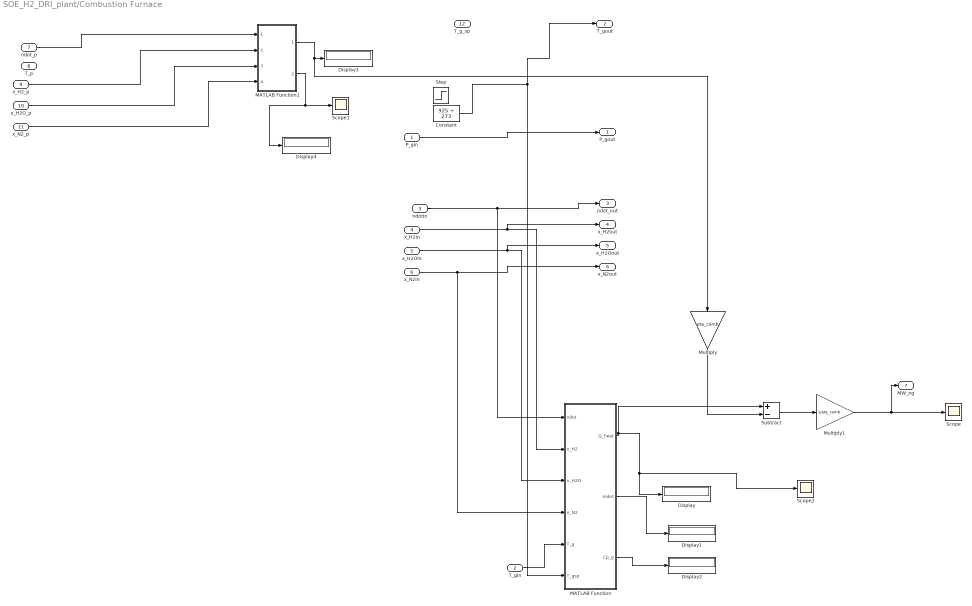
== system SOE_H2_DRI_plant/Combustion Furnace ==
  P_gin : Inport
  T_gin : Inport  Port=2
  ndotin : Inport  Port=3
  x_H2in : Inport  Port=4
  x_H2Oin : Inport  Port=5
  x_N2in : Inport  Port=6
  ndot_p : Inport  Port=7
  T_p : Inport  Port=8
  x_H2_p : Inport  Port=9
  x_H2O_p : Inport  Port=10
  x_N2_p : Inport  Port=11
  T_g_sp : Inport  Port=12
  Constant : Constant  Value=925 + 273
  Display{,1..4} (5 alike) : Display
  MATLAB Function : MATLAB Function  TreatAsAtomicUnit=on
  MATLAB Function1 : MATLAB Function  TreatAsAtomicUnit=on
  Multiply : Gain  Gain=eta_comb
  Multiply1 : Gain  Gain=1/eta_comb
  Scope : Scope
  Scope1 : Scope
  Scope2 : Scope
  Step : Step  Time=3600*24*2  Before=925+273  After=950+273  SampleTime=0
  Subtract : Sum  Inputs=+-
  P_gout : Outport
  T_gout : Outport  Port=2
  ndot_out : Outport  Port=3
  x_H2out : Outport  Port=4
  x_H2Oout : Outport  Port=5
  x_N2out : Outport  Port=6
  MW_ng : Outport  Port=7
  wires:
  P_gin/1 -> P_gout/1
  x_H2in/1 -> MATLAB Function/2(x_H2), x_H2out/1
  x_H2Oin/1 -> MATLAB Function/3(x_H2O), x_H2Oout/1
  x_N2in/1 -> MATLAB Function/4(x_N2), x_N2out/1
  ndotin/1 -> MATLAB Function/1(ndot), ndot_out/1
  Constant/1 -> MATLAB Function/6(T_gsp), T_gout/1
  x_H2_p/1 -> MATLAB Function1/2(x_H2_p)
  x_H2O_p/1 -> MATLAB Function1/3(x_H2O_p)
  x_N2_p/1 -> MATLAB Function1/4(x_N2_p)
  T_gin/1 -> MATLAB Function/5(T_g)
  MATLAB Function/2(mdot) -> Display1/1
  MATLAB Function/3(Cp_g) -> Display2/1
  ndot_p/1 -> MATLAB Function1/1(ndot_p)
  MATLAB Function1/1(Q_purge) -> Multiply/1, Display3/1
  MATLAB Function/1(Q_heat) -> Subtract/1, Scope2/1, Display/1
  Subtract/1 -> Multiply1/1
  Multiply/1 -> Subtract/2
  Multiply1/1 -> MW_ng/1, Scope/1
  MATLAB Function1/2(mdot_p) -> Scope1/1, Display4/1

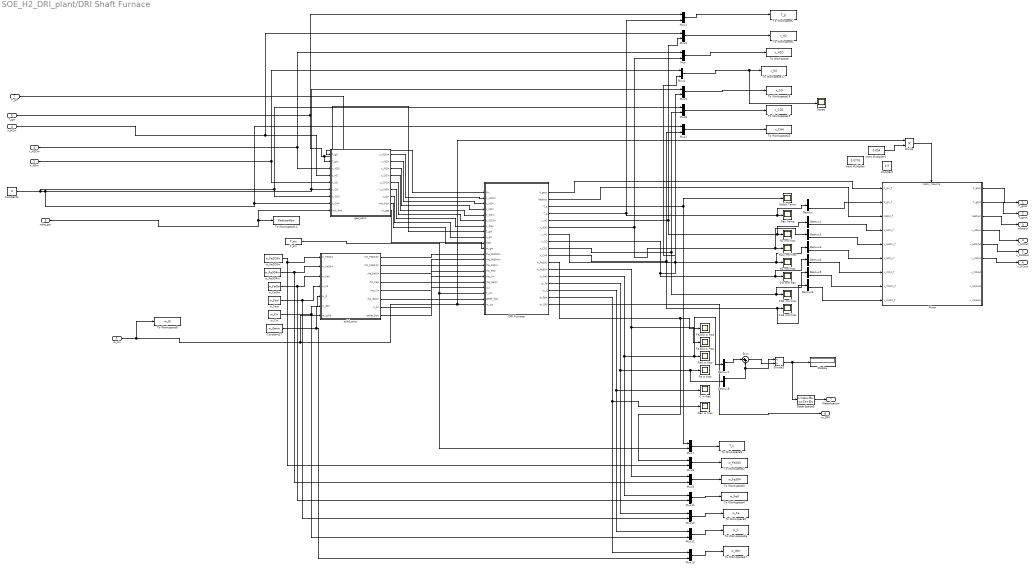
== system SOE_H2_DRI_plant/DRI Shaft Furnace ==
  m_sin : Inport
  x_N2in : Inport  Port=2
  x_H2Oin : Inport  Port=3
  x_H2in : Inport  Port=4
  ndot_gin : Inport  Port=5
  T_gin : Inport  Port=6
  P_gin : Inport  Port=7
  C w frac : Scope
  CH4 mol frac : Scope
  CO mol frac : Scope
  CO2 mol frac : Scope
  Constant : Constant  Value=3.5
  Constant1 : Constant  Value=0
  Constant17 : Constant  Value=w_Ganin
  DRI Furnace : Subsystem
      mask Display: image('discretization.png');
  Demux{,1..6} (7 alike) : Demux  Outputs=[n_furnace-1 1]
  Demux7 : Demux  Outputs=[1 n_furnace-1]
  Demux8 : Demux  Outputs=[1 n_furnace-1]
  Display : Display
  Divide : Product  Inputs=**
  Divide3 : Product  Inputs=*/
  Fe w frac : Scope
  Fe2O3 w frac : Scope
  Fe3O4 w frac : Scope
  FeO w frac : Scope
  Gan w frac : Scope
  Gas Temp : Scope
  H2 mol frac : Scope
  H2O mol frac : Scope
  Inert Multiplier : Constant  Value=0.0776
  Inert Multiplier1 : Constant  Value=0.054
  Mixer : Subsystem
      settings: PortSchema="{\"entries\":[{\"content\":{\"sides\":[{\"content\":{\"connectorIds\":[\"In1\",\"In2\",\"In3\",\"In4\",\"In5\",\"In6\",\"In7\",\"In8\",\"In9\"]},\"type\":\"ConnectorPlacement.EquallySpacedRectSide\",\"uuid\":\"655e84cb-69cf-4761-b101-58ad49abce33\"},{\"content\":{\"connectorIds\":[\"Out1\",\"Out2\",\"Out3\",\"Out4\",\"Out5\",\"Out6\",\"Out7\",\"Out8\",\"Out9\"],\"side\":\"RIGHT\"},\"type\":\"ConnectorPlacement.EquallySpacedRectSide\",\"uuid\":\"c22001c3-4fe9-4ca1-8f86-27c8b9cf3215\"},{\"content\":{\"connectorIds\":[\"In10\"],\"side\":\"TOP\"},\"type\":\"ConnectorPlacement.EquallySpacedRectSide\",\"uuid\":\"85460019-312d-4580-833a-9195b760a2b2\"}]},\"type\":\"ConnectorPlacement.EquallySpacedConnector\",\"uuid\":\"a09837c3-5ba4-4c5d-b1a3-49fb7b0895f7\"}],\"packageUris\":[\"http://schema.mathworks.com/mf0/Connector/R2020b\"],\"version\":\"1.0\"}"
      mask Display: image('Mixer.drawio.png');
  Mux{,1..13} (14 alike) : Mux  Inputs=2
  N2 mol frac : Scope
  Scope : Scope
  Solids Temp : Scope
  State-Space5 : StateSpace  A=-1/(tau)  B=1/(tau)  D=0  InitialCondition=0.95
  Sum : Sum  Inputs=|++
  T_sin : Constant  Value=T_sin
  To Workspace : ToWorkspace  VariableName=x_H2O  SaveFormat=Timeseries  SampleTime=-1
  To Workspace1 : ToWorkspace  VariableName=x_H2  SaveFormat=Timeseries  SampleTime=-1
  To Workspace11 : ToWorkspace  VariableName=Reducerflow  SaveFormat=Timeseries  SampleTime=-1
  To Workspace17 : ToWorkspace  VariableName=x_N2  SaveFormat=Timeseries  SampleTime=-1
  To Workspace18 : ToWorkspace  VariableName=x_CO  SaveFormat=Timeseries  SampleTime=-1
  To Workspace19 : ToWorkspace  VariableName=x_CO2  SaveFormat=Timeseries  SampleTime=-1
  To Workspace2 : ToWorkspace  VariableName=w_Fe2O3  SaveFormat=Timeseries  SampleTime=-1
  To Workspace23 : ToWorkspace  VariableName=x_CH4  SaveFormat=Timeseries  SampleTime=-1
  To Workspace26 : ToWorkspace  VariableName=w_C  SaveFormat=Timeseries  SampleTime=-1
  To Workspace27 : ToWorkspace  VariableName=w_Gan  SaveFormat=Timeseries  SampleTime=-1
  To Workspace3 : ToWorkspace  VariableName=w_Fe3O4  SaveFormat=Timeseries  SampleTime=-1
  To Workspace4 : ToWorkspace  VariableName=w_FeO  SaveFormat=Timeseries  SampleTime=-1
  To Workspace5 : ToWorkspace  VariableName=w_Fe  SaveFormat=Timeseries  SampleTime=-1
  To Workspace6 : ToWorkspace  VariableName=T_s  SaveFormat=Timeseries  SampleTime=-1
  To Workspace7 : ToWorkspace  VariableName=T_g  SaveFormat=Timeseries  SampleTime=-1
  To Workspace8 : ToWorkspace  VariableName=m_IO  SaveFormat=Timeseries  SampleTime=-1
  gas_conc : MATLAB Function  TreatAsAtomicUnit=on
  solid_conc : MATLAB Function  TreatAsAtomicUnit=on
  w_Cin : Constant  Value=w_Cin
  w_Fe2O3in : Constant  Value=w_Fe2O3in
  w_Fe3O4in : Constant  Value=w_Fe3O4in
  w_FeOin : Constant  Value=w_FeOin
  w_Fein : Constant  Value=w_Fein
  P_gout : Outport
  T_gout : Outport  Port=2
  ndotout : Outport  Port=3
  x_H2out : Outport  Port=4
  x_H2Oout : Outport  Port=5
  x_N2out : Outport  Port=6
  Mettalization : Outport  Port=7
  m_DRI : Outport  Port=8
  wires:
  DRI Furnace/7(x_N2) -> Demux3/1, N2 mol frac/1, Mux4/2
  solid_conc/8(pellet_flow) -> DRI Furnace/20(pellet_flow)
  gas_conc/2(c_H2in) -> DRI Furnace/3(c_H2in)
  DRI Furnace/5(x_H2) -> Mux3/2, Demux1/1, H2 mol frac/1
  w_Fe3O4in/1 -> Mux9/2, solid_conc/2(w_Fe3O4)
  gas_conc/3(c_N2in) -> DRI Furnace/4(c_N2in)
  gas_conc/4(c_COin) -> DRI Furnace/5(c_COin)
  w_FeOin/1 -> Mux11/2, solid_conc/3(w_FeO)
  P_gin/1 -> gas_conc/1(P_gin), DRI Furnace/1(Pin)
  x_H2in/1 -> gas_conc/4(x_H2), Mux3/1
  T_sin/1 -> DRI Furnace/19(T_sin), Mux7/2
  DRI Furnace/3(T_s) -> Solids Temp/1, Mux7/1
  Constant1/1 -> gas_conc/7(x_CO2), Mux6/1, Mux2/1, gas_conc/8(x_CH4), Mux5/1, gas_conc/6(x_CO)
  solid_conc/4(rho_Fein) -> DRI Furnace/15(rho_Fein)
  solid_conc/5(rho_Cin) -> DRI Furnace/16(rho_Cin)
  m_sin/1 -> To Workspace8/1, solid_conc/7(m_solid), Divide/1, DRI Furnace/21(m_sin)
  DRI Furnace/9(x_CO2) -> Mux6/2, Demux5/1, CO2 mol frac/1
  ndot_gin/1 -> gas_conc/9("mol_flow "), To Workspace11/1
  solid_conc/3(rho_FeOin) -> DRI Furnace/14(rho_FeOin)
  gas_conc/8(mol_flow) -> DRI Furnace/10(ndot)
  Mux12/1 -> To Workspace26/1
  DRI Furnace/8(x_CO) -> Demux4/1, CO mol frac/1, Mux5/2
  DRI Furnace/15(w_C) -> C w frac/1, Mux12/1
  w_Cin/1 -> solid_conc/5(w_C), Mux12/2
  gas_conc/7(u_gin) -> DRI Furnace/9(u_gin)
  DRI Furnace/13(w_FeO) -> Demux7/1, FeO w frac/1, Mux11/1
  Mux13/1 -> To Workspace27/1
  DRI Furnace/14(w_Fe) -> Demux8/1, Fe w frac/1, Mux10/1
  Mux8/1 -> To Workspace2/1
  DRI Furnace/10(x_CH4) -> Mux2/2, Demux6/1, CH4 mol frac/1
  Mux4/1 -> Scope/1, To Workspace17/1
  T_gin/1 -> DRI Furnace/8(T_gin), gas_conc/2(T_gin), Mux1/1
  gas_conc/5(c_CO2in) -> DRI Furnace/6(c_CO2in)
  w_Fe2O3in/1 -> solid_conc/1(w_Fe2O3), Mux8/2
  solid_conc/6(rho_Ganin) -> DRI Furnace/17(rho_Ganin)
  Mux/1 -> To Workspace/1
  Mux11/1 -> To Workspace4/1
  Mux10/1 -> To Workspace5/1
  DRI Furnace/6(x_H2O) -> Mux/2, Demux2/1, H2O mol frac/1
  solid_conc/7(u_sin) -> DRI Furnace/18(u_s)
  DRI Furnace/4(T_g) -> Mux1/2, Demux/1, Gas Temp/1
  DRI Furnace/16(w_Gan) -> Gan w frac/1, Mux13/1
  solid_conc/1(rho_Fe2O3in) -> DRI Furnace/12(rho_Fe2O3in)
  DRI Furnace/12(w_Fe3O4) -> Fe3O4 w frac/1, Mux9/1
  Constant17/1 -> Mux13/2, solid_conc/6(w_Gan)
  gas_conc/1(c_H2Oin) -> DRI Furnace/2(c_H2Oin)
  Mux3/1 -> To Workspace1/1
  Mux6/1 -> To Workspace19/1
  Mux1/1 -> To Workspace7/1
  Mux7/1 -> To Workspace6/1
  DRI Furnace/11(w_Fe2O3) -> Mux8/1, Fe2O3 w frac/1
  Mux2/1 -> To Workspace23/1
  w_Fein/1 -> Mux10/2, solid_conc/4(w_Fe)
  gas_conc/6(c_CH4in) -> DRI Furnace/7(c_CH4)
  Mux5/1 -> To Workspace18/1
  Mux9/1 -> To Workspace3/1
  solid_conc/2(rho_Fe3O4in) -> DRI Furnace/13(rho_Fe3O4in)
  x_N2in/1 -> gas_conc/5(x_N2), Mux4/1
  x_H2Oin/1 -> gas_conc/3(x_H2O), Mux/1
  DRI Furnace/1(P_gout) -> Mixer/1(P_gin_f)
  Demux1/2 -> Mixer/4(x_H2in_f)
  Demux2/2 -> Mixer/5(x_H2Oin_f)
  Demux4/2 -> Mixer/7(x_COin_f)
  Demux5/2 -> Mixer/8(x_CO2in_f)
  Demux6/2 -> Mixer/9(x_CH4in_f)
  gas_conc/9(m_gas) -> DRI Furnace/11(m_gin)
  Mixer/1(P_gout) -> P_gout/1
  Mixer/2(T_gout) -> T_gout/1
  Mixer/5(x_H2Oout) -> x_H2Oout/1
  Mixer/6(x_N2out) -> x_N2out/1
  Demux/2 -> Mixer/2(T_gin_f)
  Divide/1 -> Mixer/10(ndotin_N2extra)
  DRI Furnace/2(ndotout) -> Mixer/3(ndotin_f)
  Demux3/2 -> Mixer/6(x_N2in_f)
  Mixer/3(ndotout) -> ndotout/1
  Mixer/4(x_H2out) -> x_H2out/1
  Inert Multiplier1/1 -> Divide/2
  Sum/1 -> Divide3/2
  Demux7/1 -> Sum/1
  Demux8/1 -> Divide3/1, Sum/2
  Divide3/1 -> State-Space5/1, Display/1
  State-Space5/1 -> Mettalization/1
  DRI Furnace/17(m_DRI) -> m_DRI/1

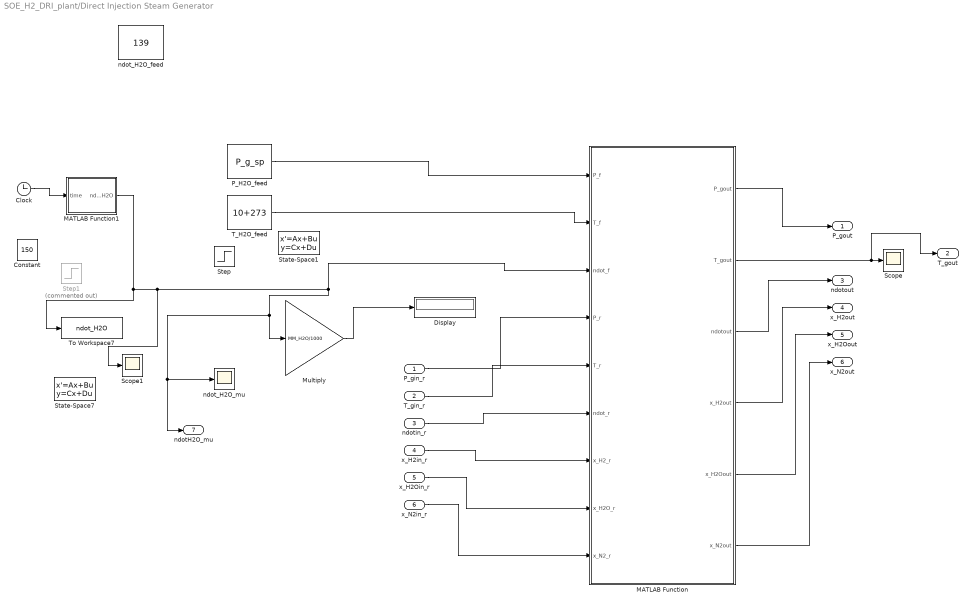
== system SOE_H2_DRI_plant/Direct Injection Steam Generator ==
  P_gin_r : Inport
  T_gin_r : Inport  Port=2
  ndotin_r : Inport  Port=3
  x_H2in_r : Inport  Port=4
  x_H2Oin_r : Inport  Port=5
  x_N2in_r : Inport  Port=6
  Clock : Clock
  Constant : Constant  Value=150
  Display : Display
  MATLAB Function : MATLAB Function  TreatAsAtomicUnit=on
  MATLAB Function1 : MATLAB Function  TreatAsAtomicUnit=on
  Multiply : Gain  Gain=MM_H2O/1000
  P_H2O_feed : Constant  Value=P_g_sp
  Scope : Scope
  Scope1 : Scope
  State-Space1 : StateSpace  A=-1/(3600*24)  B=1/(3600*24)  D=0  InitialCondition=139
  State-Space7 : StateSpace  A=-1/(3600*12)  B=1/(3600*12)  D=0  InitialCondition=100
  Step : Step  Time=3600*6  Before=139  After=139  SampleTime=0
  Step1 : Step  Commented=on  Time=3600*24*2  Before=100  After=ndot_H2O_feed  SampleTime=0
  T_H2O_feed : Constant  Value=10+273
  To Workspace7 : ToWorkspace  VariableName=ndot_H2O  SaveFormat=Timeseries  SampleTime=-1
  ndot_H2O_feed : Constant  Value=139
  ndot_H2O_mu : Scope
  P_gout : Outport
  T_gout : Outport  Port=2
  ndotout : Outport  Port=3
  x_H2out : Outport  Port=4
  x_H2Oout : Outport  Port=5
  x_N2out : Outport  Port=6
  ndotH2O_mu : Outport  Port=7
  wires:
  MATLAB Function/1(P_gout) -> P_gout/1
  MATLAB Function/3(ndotout) -> ndotout/1
  MATLAB Function/4(x_H2out) -> x_H2out/1
  MATLAB Function/5(x_H2Oout) -> x_H2Oout/1
  MATLAB Function/6(x_N2out) -> x_N2out/1
  P_gin_r/1 -> MATLAB Function/4(P_r)
  T_gin_r/1 -> MATLAB Function/5(T_r)
  ndotin_r/1 -> MATLAB Function/6(ndot_r)
  x_H2in_r/1 -> MATLAB Function/7(x_H2_r)
  x_H2Oin_r/1 -> MATLAB Function/8(x_H2O_r)
  x_N2in_r/1 -> MATLAB Function/9(x_N2_r)
  MATLAB Function/2(T_gout) -> T_gout/1, Scope/1
  T_H2O_feed/1 -> MATLAB Function/2(T_f)
  P_H2O_feed/1 -> MATLAB Function/1(P_f)
  Multiply/1 -> Display/1
  Clock/1 -> MATLAB Function1/1(time)
  MATLAB Function1/1(ndot_H2O) -> To Workspace7/1, Scope1/1, MATLAB Function/3(ndot_f), ndot_H2O_mu/1, ndotH2O_mu/1, Multiply/1

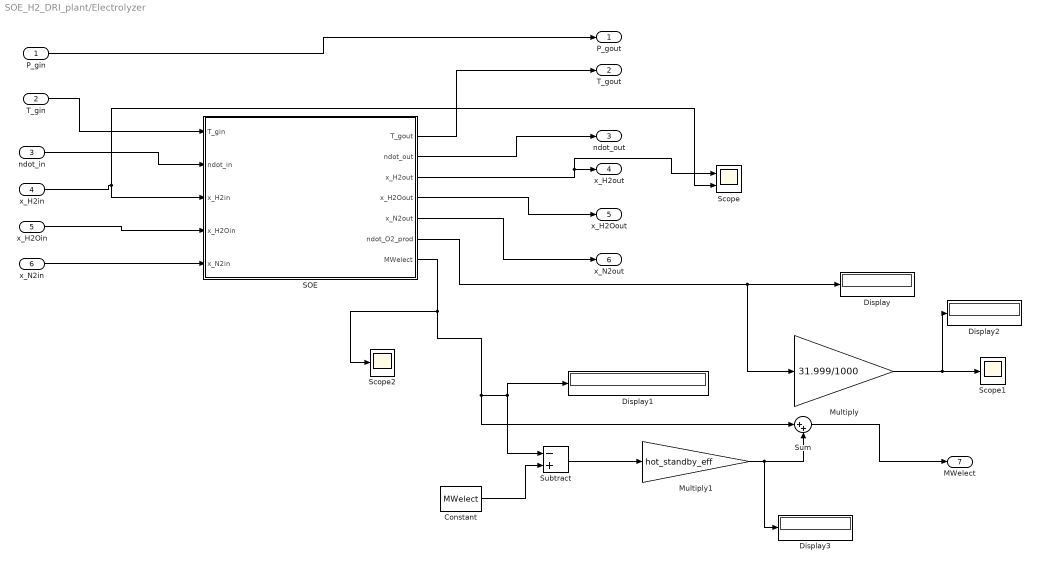
== system SOE_H2_DRI_plant/Electrolyzer ==
  P_gin : Inport
  T_gin : Inport  Port=2
  ndot_in : Inport  Port=3
  x_H2in : Inport  Port=4
  x_H2Oin : Inport  Port=5
  x_N2in : Inport  Port=6
  Constant : Constant  Value=MWelect
  Display{,1..3} (4 alike) : Display
  Multiply : Gain  Gain=31.999/1000
  Multiply1 : Gain  Gain=hot_standby_eff
  SOE : MATLAB Function  TreatAsAtomicUnit=on
  Scope : Scope  NumInputPorts=2
  Scope1 : Scope
  Scope2 : Scope
  Subtract : Sum  Inputs=-+
  Sum : Sum  Inputs=|++
  P_gout : Outport
  T_gout : Outport  Port=2
  ndot_out : Outport  Port=3
  x_H2out : Outport  Port=4
  x_H2Oout : Outport  Port=5
  x_N2out : Outport  Port=6
  MWelect : Outport  Port=7
  wires:
  SOE/1(T_gout) -> T_gout/1
  x_N2in/1 -> SOE/5(x_N2in)
  x_H2Oin/1 -> SOE/4(x_H2Oin)
  x_H2in/1 -> Scope/2, SOE/3(x_H2in)
  ndot_in/1 -> SOE/2(ndot_in)
  T_gin/1 -> SOE/1(T_gin)
  P_gin/1 -> P_gout/1
  SOE/2(ndot_out) -> ndot_out/1
  SOE/3(x_H2out) -> Scope/1, x_H2out/1
  SOE/4(x_H2Oout) -> x_H2Oout/1
  SOE/5(x_N2out) -> x_N2out/1
  SOE/7(MWelect) -> Scope2/1, Sum/1, Display1/1, Subtract/1
  Multiply/1 -> Display2/1, Scope1/1
  SOE/6(ndot_O2_prod) -> Multiply/1, Display/1
  Constant/1 -> Subtract/2
  Subtract/1 -> Multiply1/1
  Multiply1/1 -> Sum/2, Display3/1
  Sum/1 -> MWelect/1

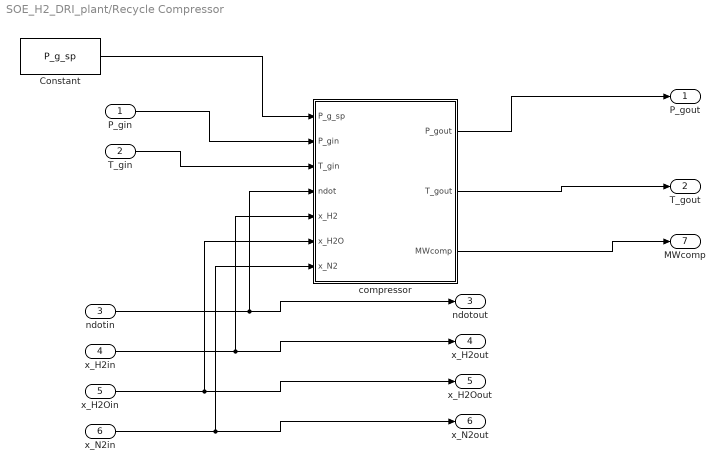
== system SOE_H2_DRI_plant/Recycle Compressor ==
  P_gin : Inport
  T_gin : Inport  Port=2
  ndotin : Inport  Port=3
  x_H2in : Inport  Port=4
  x_H2Oin : Inport  Port=5
  x_N2in : Inport  Port=6
  Constant : Constant  Value=P_g_sp
  compressor : MATLAB Function  TreatAsAtomicUnit=on
  P_gout : Outport
  T_gout : Outport  Port=2
  ndotout : Outport  Port=3
  x_H2out : Outport  Port=4
  x_H2Oout : Outport  Port=5
  x_N2out : Outport  Port=6
  MWcomp : Outport  Port=7
  wires:
  x_H2in/1 -> compressor/5(x_H2), x_H2out/1
  x_H2Oin/1 -> compressor/6(x_H2O), x_H2Oout/1
  x_N2in/1 -> compressor/7(x_N2), x_N2out/1
  compressor/1(P_gout) -> P_gout/1
  compressor/2(T_gout) -> T_gout/1
  P_gin/1 -> compressor/2(P_gin)
  T_gin/1 -> compressor/3(T_gin)
  ndotin/1 -> compressor/4(ndot), ndotout/1
  Constant/1 -> compressor/1(P_g_sp)
  compressor/3(MWcomp) -> MWcomp/1

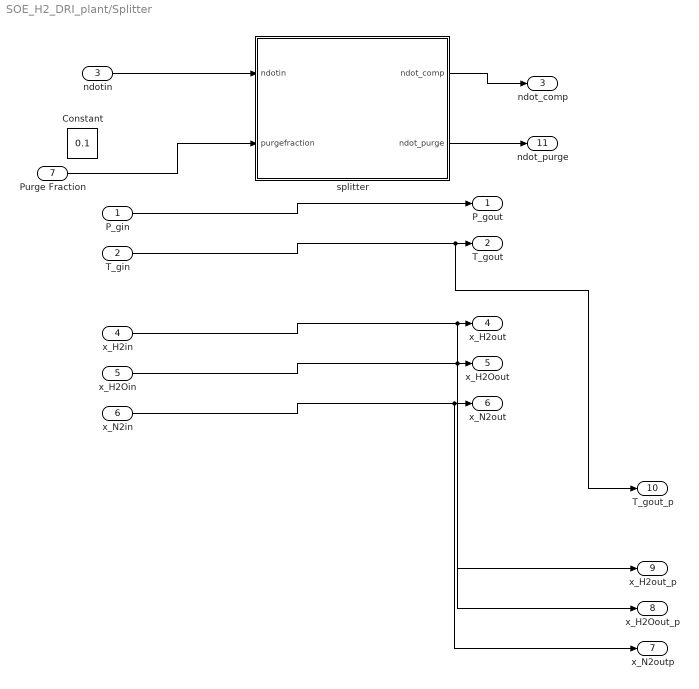
== system SOE_H2_DRI_plant/Splitter ==
  P_gin : Inport
  T_gin : Inport  Port=2
  ndotin : Inport  Port=3
  x_H2in : Inport  Port=4
  x_H2Oin : Inport  Port=5
  x_N2in : Inport  Port=6
  Purge Fraction : Inport  Port=7
  Constant : Constant  Value=0.1
  splitter : MATLAB Function  TreatAsAtomicUnit=on
  P_gout : Outport
  T_gout : Outport  Port=2
  ndot_comp : Outport  Port=3
  x_H2out : Outport  Port=4
  x_H2Oout : Outport  Port=5
  x_N2out : Outport  Port=6
  x_N2outp : Outport  Port=7
  x_H2Oout_p : Outport  Port=8
  x_H2out_p : Outport  Port=9
  T_gout_p : Outport  Port=10
  ndot_purge : Outport  Port=11
  wires:
  ndotin/1 -> splitter/1(ndotin)
  P_gin/1 -> P_gout/1
  T_gin/1 -> T_gout_p/1, T_gout/1
  x_H2in/1 -> x_H2out_p/1, x_H2out/1
  x_H2Oin/1 -> x_H2Oout_p/1, x_H2Oout/1
  splitter/1(ndot_comp) -> ndot_comp/1
  Purge Fraction/1 -> splitter/2(purgefraction)
  splitter/2(ndot_purge) -> ndot_purge/1
  x_N2in/1 -> x_N2outp/1, x_N2out/1

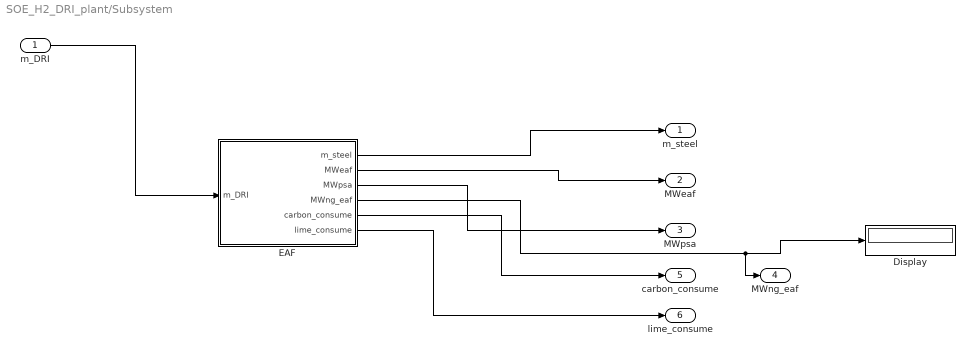
== system SOE_H2_DRI_plant/Subsystem ==
  m_DRI : Inport
  Display : Display
  EAF : MATLAB Function  TreatAsAtomicUnit=on
  m_steel : Outport
  MWeaf : Outport  Port=2
  MWpsa : Outport  Port=3
  MWng_eaf : Outport  Port=4
  carbon_consume : Outport  Port=5
  lime_consume : Outport  Port=6
  wires:
  EAF/1(m_steel) -> m_steel/1
  m_DRI/1 -> EAF/1(m_DRI)
  EAF/2(MWeaf) -> MWeaf/1
  EAF/3(MWpsa) -> MWpsa/1
  EAF/5(carbon_consume) -> carbon_consume/1
  EAF/6(lime_consume) -> lime_consume/1
  EAF/4(MWng_eaf) -> MWng_eaf/1, Display/1

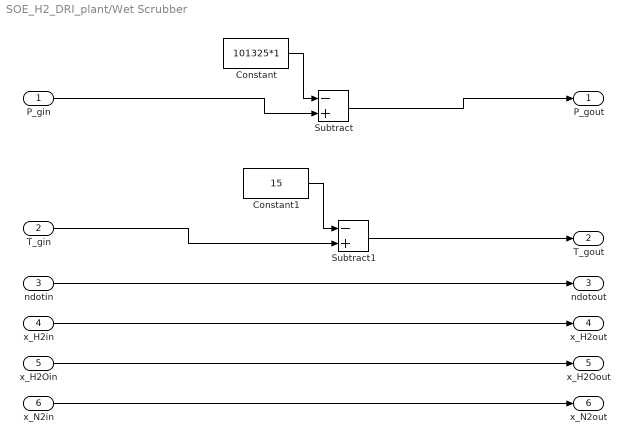
== system SOE_H2_DRI_plant/Wet Scrubber ==
  P_gin : Inport
  T_gin : Inport  Port=2
  ndotin : Inport  Port=3
  x_H2in : Inport  Port=4
  x_H2Oin : Inport  Port=5
  x_N2in : Inport  Port=6
  Constant : Constant  Value=101325*1
  Constant1 : Constant  Value=15
  Subtract : Sum  Inputs=-+
  Subtract1 : Sum  Inputs=-+
  P_gout : Outport
  T_gout : Outport  Port=2
  ndotout : Outport  Port=3
  x_H2out : Outport  Port=4
  x_H2Oout : Outport  Port=5
  x_N2out : Outport  Port=6
  wires:
  P_gin/1 -> Subtract/2
  ndotin/1 -> ndotout/1
  x_H2in/1 -> x_H2out/1
  x_H2Oin/1 -> x_H2Oout/1
  x_N2in/1 -> x_N2out/1
  Subtract/1 -> P_gout/1
  Constant/1 -> Subtract/1
  Constant1/1 -> Subtract1/1
  T_gin/1 -> Subtract1/2
  Subtract1/1 -> T_gout/1
